simulink model "Stoplight"  (R2020a)
settings: Solver=VariableStepAuto  StartTime=0.0  StopTime=inf  RelTol=1e-3
libraries: dspnetwork x21, sldrtlib x1
settings Model: Creator=brandon  LastModifiedBy=brandon

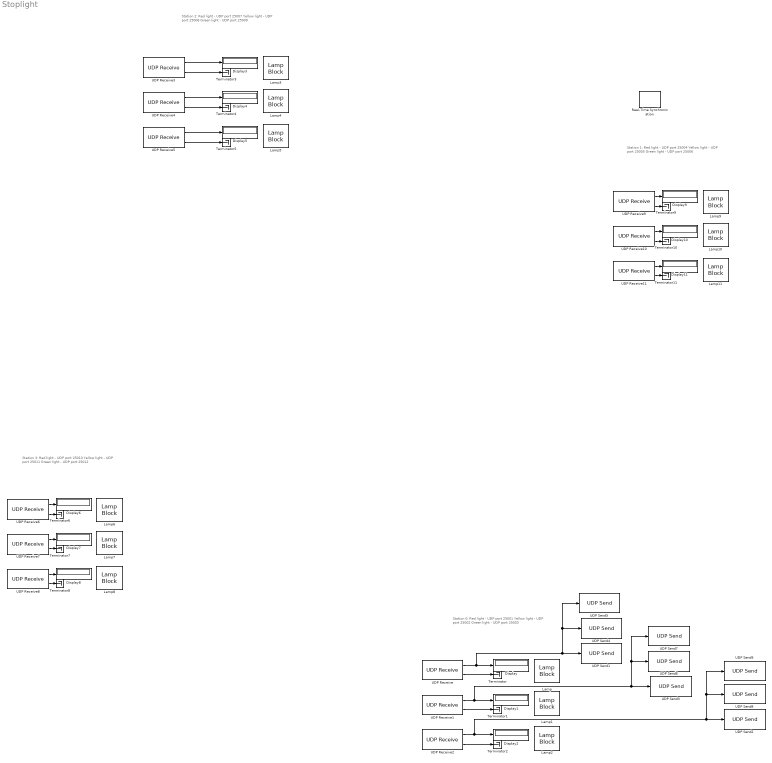
== system Stoplight ==
  note: Station 0:
      | Red light - UDP port 25001
      | Yellow light - UDP port 25002
      | Green light - UDP port 25003
  note: Station 1:
      | Red light - UDP port 25004
      | Yellow light - UDP port 25005
      | Green light - UDP port 25006
  note: Station 2:
      | Red light - UDP port 25007
      | Yellow light - UDP port 25008
      | Green light - UDP port 25009
  note: Station 3:
      | Red light - UDP port 25010
      | Yellow light - UDP port 25011
      | Green light - UDP port 25012
  Display{,1..11} (12 alike) : Display
  Lamp{,1..11} (12 alike) : LampBlock  LabelPosition=Hide
  Real-Time Synchronization : sldrtlib/Real-Time Synchronization  SampleTime=0.1  MaxMissedTicks=1000000  ShowMissedTicks=off  YieldWhenWaiting=off
  Terminator{,1..11} (12 alike) : Terminator
  UDP Receive : dspnetwork/UDP Receive  localURL='0.0.0.0'  localPort=25001  remoteURL='0.0.0.0'  remotePort=-1  recvBufferSize=2  dims=1  signalDatatype=uint16  isComplex=off  isVarSize=off  showBlockingTime=off  blockingTime=0  sampletime=0.1  blockPlatform=[]
  UDP Receive1 : dspnetwork/UDP Receive  localURL='0.0.0.0'  localPort=25002  remoteURL='0.0.0.0'  remotePort=-1  recvBufferSize=2  dims=1  signalDatatype=uint16  isComplex=off  isVarSize=off  showBlockingTime=off  blockingTime=0  sampletime=0.1  blockPlatform=[]
  UDP Receive10 : dspnetwork/UDP Receive  localURL='0.0.0.0'  localPort=25005  remoteURL='0.0.0.0'  remotePort=-1  recvBufferSize=2  dims=1  signalDatatype=uint16  isComplex=off  isVarSize=off  showBlockingTime=off  blockingTime=0  sampletime=0.1  blockPlatform=[]
  UDP Receive11 : dspnetwork/UDP Receive  localURL='0.0.0.0'  localPort=25006  remoteURL='0.0.0.0'  remotePort=-1  recvBufferSize=2  dims=1  signalDatatype=uint16  isComplex=off  isVarSize=off  showBlockingTime=off  blockingTime=0  sampletime=0.1  blockPlatform=[]
  UDP Receive2 : dspnetwork/UDP Receive  localURL='0.0.0.0'  localPort=25003  remoteURL='0.0.0.0'  remotePort=-1  recvBufferSize=2  dims=1  signalDatatype=uint16  isComplex=off  isVarSize=off  showBlockingTime=off  blockingTime=0  sampletime=0.1  blockPlatform=[]
  UDP Receive3 : dspnetwork/UDP Receive  localURL='0.0.0.0'  localPort=25007  remoteURL='0.0.0.0'  remotePort=-1  recvBufferSize=2  dims=1  signalDatatype=uint16  isComplex=off  isVarSize=off  showBlockingTime=off  blockingTime=0  sampletime=0.1  blockPlatform=[]
  UDP Receive4 : dspnetwork/UDP Receive  localURL='0.0.0.0'  localPort=25008  remoteURL='0.0.0.0'  remotePort=-1  recvBufferSize=2  dims=1  signalDatatype=uint16  isComplex=off  isVarSize=off  showBlockingTime=off  blockingTime=0  sampletime=0.1  blockPlatform=[]
  UDP Receive5 : dspnetwork/UDP Receive  localURL='0.0.0.0'  localPort=25009  remoteURL='0.0.0.0'  remotePort=-1  recvBufferSize=2  dims=1  signalDatatype=uint16  isComplex=off  isVarSize=off  showBlockingTime=off  blockingTime=0  sampletime=0.1  blockPlatform=[]
  UDP Receive6 : dspnetwork/UDP Receive  localURL='0.0.0.0'  localPort=25010  remoteURL='0.0.0.0'  remotePort=-1  recvBufferSize=2  dims=1  signalDatatype=uint16  isComplex=off  isVarSize=off  showBlockingTime=off  blockingTime=0  sampletime=0.1  blockPlatform=[]
  UDP Receive7 : dspnetwork/UDP Receive  localURL='0.0.0.0'  localPort=25011  remoteURL='0.0.0.0'  remotePort=-1  recvBufferSize=2  dims=1  signalDatatype=uint16  isComplex=off  isVarSize=off  showBlockingTime=off  blockingTime=0  sampletime=0.1  blockPlatform=[]
  UDP Receive8 : dspnetwork/UDP Receive  localURL='0.0.0.0'  localPort=25012  remoteURL='0.0.0.0'  remotePort=-1  recvBufferSize=2  dims=1  signalDatatype=uint16  isComplex=off  isVarSize=off  showBlockingTime=off  blockingTime=0  sampletime=0.1  blockPlatform=[]
  UDP Receive9 : dspnetwork/UDP Receive  localURL='0.0.0.0'  localPort=25004  remoteURL='0.0.0.0'  remotePort=-1  recvBufferSize=2  dims=1  signalDatatype=uint16  isComplex=off  isVarSize=off  showBlockingTime=off  blockingTime=0  sampletime=0.1  blockPlatform=[]
  UDP Send1 : dspnetwork/UDP Send  remoteURL='192.168.88.34'  remotePort=26004  localURL='0.0.0.0'  localPortSource=Automatically determine  localPort=-1  sendBufferSize=2  sampletime=-1  blockPlatform=[]  separateLengthPort=0
  UDP Send2 : dspnetwork/UDP Send  remoteURL='192.168.88.34'  remotePort=26006  localURL='0.0.0.0'  localPortSource=Automatically determine  localPort=-1  sendBufferSize=2  sampletime=-1  blockPlatform=[]  separateLengthPort=0
  UDP Send3 : dspnetwork/UDP Send  remoteURL='192.168.88.34'  remotePort=26005  localURL='0.0.0.0'  localPortSource=Automatically determine  localPort=-1  sendBufferSize=2  sampletime=-1  blockPlatform=[]  separateLengthPort=0
  UDP Send4 : dspnetwork/UDP Send  remoteURL='192.168.88.34'  remotePort=26001  localURL='0.0.0.0'  localPortSource=Automatically determine  localPort=-1  sendBufferSize=2  sampletime=-1  blockPlatform=[]  separateLengthPort=0
  UDP Send5 : dspnetwork/UDP Send  remoteURL='192.168.88.34'  remotePort=26007  localURL='0.0.0.0'  localPortSource=Automatically determine  localPort=-1  sendBufferSize=2  sampletime=-1  blockPlatform=[]  separateLengthPort=0
  UDP Send6 : dspnetwork/UDP Send  remoteURL='192.168.88.34'  remotePort=26002  localURL='0.0.0.0'  localPortSource=Automatically determine  localPort=-1  sendBufferSize=2  sampletime=-1  blockPlatform=[]  separateLengthPort=0
  UDP Send7 : dspnetwork/UDP Send  remoteURL='192.168.88.34'  remotePort=26008  localURL='0.0.0.0'  localPortSource=Automatically determine  localPort=-1  sendBufferSize=2  sampletime=-1  blockPlatform=[]  separateLengthPort=0
  UDP Send8 : dspnetwork/UDP Send  remoteURL='192.168.88.34'  remotePort=26003  localURL='0.0.0.0'  localPortSource=Automatically determine  localPort=-1  sendBufferSize=2  sampletime=-1  blockPlatform=[]  separateLengthPort=0
  UDP Send9 : dspnetwork/UDP Send  remoteURL='192.168.88.34'  remotePort=26009  localURL='0.0.0.0'  localPortSource=Automatically determine  localPort=-1  sendBufferSize=2  sampletime=-1  blockPlatform=[]  separateLengthPort=0
  wires:
  UDP Receive/2 -> Terminator/1
  UDP Receive1/2 -> Terminator1/1
  UDP Receive2/2 -> Terminator2/1
  UDP Receive/1 -> UDP Send5/1, UDP Send4/1, UDP Send1/1, Display/1
  UDP Receive1/1 -> UDP Send7/1, UDP Send6/1, UDP Send3/1, Display1/1
  UDP Receive2/1 -> UDP Send9/1, UDP Send8/1, UDP Send2/1, Display2/1
  UDP Receive5/2 -> Terminator5/1
  UDP Receive4/1 -> Display4/1
  UDP Receive4/2 -> Terminator4/1
  UDP Receive5/1 -> Display5/1
  UDP Receive3/1 -> Display3/1
  UDP Receive3/2 -> Terminator3/1
  UDP Receive8/2 -> Terminator8/1
  UDP Receive7/1 -> Display7/1
  UDP Receive7/2 -> Terminator7/1
  UDP Receive8/1 -> Display8/1
  UDP Receive6/1 -> Display6/1
  UDP Receive6/2 -> Terminator6/1
  UDP Receive11/2 -> Terminator11/1
  UDP Receive10/1 -> Display10/1
  UDP Receive10/2 -> Terminator10/1
  UDP Receive11/1 -> Display11/1
  UDP Receive9/1 -> Display9/1
  UDP Receive9/2 -> Terminator9/1
